simulink model "VCU_Final_Rev5"  (R2019b)
settings: Solver=FixedStepDiscrete  StartTime=0.0  StopTime=10.0  FixedStep=0.001  RelTol=1e-3  EnableMultiTasking=on
InitFcn:
  | EcoCoder_PreCheckLic();
libraries: CoderSF_BSW_Libs x68, SF_CanService_Libs x13
settings Model: Creator=andif  LastModifiedBy=andif
settings DataIOCC: SaveFormat=Structure  SignalLoggingSaveFormat=ModelDataLogs  SaveOutput=off  SignalLogging=off  DSMLogging=off  SaveTime=off  ReturnWorkspaceOutputs=off
settings OptimizationCC: DefaultParameterBehavior=Inlined  InlineInvariantSignals=on  EnhancedBackFolding=on  StrengthReduction=on  EnableMemcpy=off  PassReuseOutputArgsAs=Individual arguments  EfficientFloat2IntCast=on  LifeSpan=1  SimCompilerOptimization=on  OptimizeBlockOrder=speed  DifferentSizesBufferReuse=on  EfficientTunableParamExpr=on
settings DebuggingCC: AlgebraicLoopMsg=none  ArtificialAlgebraicLoopMsg=none  SaveWithDisabledLinksMsg=none  SaveWithParameterizedLinksMsg=none  CheckSSInitialOutputMsg=off  UnderspecifiedInitializationDetection=Classic  SignalResolutionControl=TryResolveAll  BlockPriorityViolationMsg=error  MinStepSizeMsg=none  InheritedTsInSrcMsg=none  MultiTaskDSMMsg=none  MultiTaskCondExecSysMsg=none  MultiTaskRateTransMsg=warning  TasksWithSamePriorityMsg=none  SigSpecEnsureSampleTimeMsg=none  IntegerOverflowMsg=error  Int32ToFloatConvMsg=none  ParameterPrecisionLossMsg=none  ParameterTunabilityLossMsg=none  FixptConstOverflowMsg=error  FcnCallInpInsideContextMsg=warning  UnconnectedInputMsg=error  UnconnectedOutputMsg=error  UnconnectedLineMsg=error  FrameProcessingCompatibilityMsg=none  BusObjectLabelMismatch=none  RootOutportRequireBusObject=none  UnknownTsInhSupMsg=none  ModelReferenceDataLoggingMessage=none  SFUnusedDataAndEventsDiag=none  SFUnexpectedBacktrackingDiag=none  SFInvalidInputDataAccessInChartInitDiag=none  SFNoUnconditionalDefaultTransitionDiag=none  SFTransitionOutsideNaturalParentDiag=none  SFUnreachableExecutionPathDiag=none
settings HardwareCC: ProdBitPerPointer=32  ProdBitPerSizeT=32  ProdBitPerPtrDiffT=32  ProdLargestAtomicInteger=Long  ProdLargestAtomicFloat=Double  ProdEndianess=BigEndian  ProdWordSize=32  ProdHWDeviceType=Freescale->MPC55xx
settings ModelReferenceCC: UpdateModelReferenceTargets=Force  ModelReferenceNumInstancesAllowed=Single  PropagateSignalLabelsOutOfModel=off
settings SFSimCC: SFSimEcho=off  SimBuildMode=sf_make_clean  MATLABDynamicMemAlloc=off
settings RTWCC: Description=Ecotrons MPC5xxx  SystemTargetFile=MPC5644A.tlc  GenerateMakefile=off  TemplateMakefile=ert_default_tmf  RTWVerbose=off  RetainRTWFile=on  RTWCompilerOptimization=on
settings CodeAppCC: IgnoreCustomStorageClasses=off  OperatorAnnotations=on  CustomSymbolStrGlobalVar=$N$M  CustomSymbolStrType=$N$M  CustomSymbolStrFcn=$N$M  CustomSymbolStrFcnArg=$N$M  CustomSymbolStrBlkIO=$N$M  CustomSymbolStrMacro=$N$M
settings STFCustomTargetCC: TargetLangStandard=C99 (ISO)  CodeReplacementLibrary=ANSI_C  UtilityFuncGeneration=Shared location  MultiwordLength=256  IncludeMdlTerminateFcn=off  CombineOutputUpdateFcns=on  SuppressErrorStatus=on  ERTCustomFileBanners=on  SupportNonFinite=off  SupportComplex=off  SupportContinuousTime=off  SupportNonInlinedSFcns=off  MATLABClassNameForMDSCustomization=Simulink.SoftwareTarget.ERTCustomization  SystemTargetFile=MPC5644A.tlc
settings ERTTargetCC: TargetLangStandard=C99 (ISO)  CodeReplacementLibrary=ANSI_C  UtilityFuncGeneration=Shared location  ParMdlRefBuildCompliant=off  CompOptLevelCompliant=off  ConcurrentExecutionCompliant=off  IncludeMdlTerminateFcn=off  SuppressErrorStatus=on  SupportNonFinite=off  SupportComplex=off  RemoveResetFunc=off  ModelStepFunctionPrototypeControlCompliant=off  CPPClassGenCompliant=off  UseToolchainInfoCompliant=off  GenerateASAP2=on  InlinedParameterPlacement=NonHierarchical  ERTCustomFileTemplate=MPC5644A_file_process.tlc  ERTFilePackagingFormat=Compact  PreserveIfCondition=on  ConvertIfToSwitch=off  PreserveExternInFcnDecls=off  SuppressUnreachableDefaultCases=off

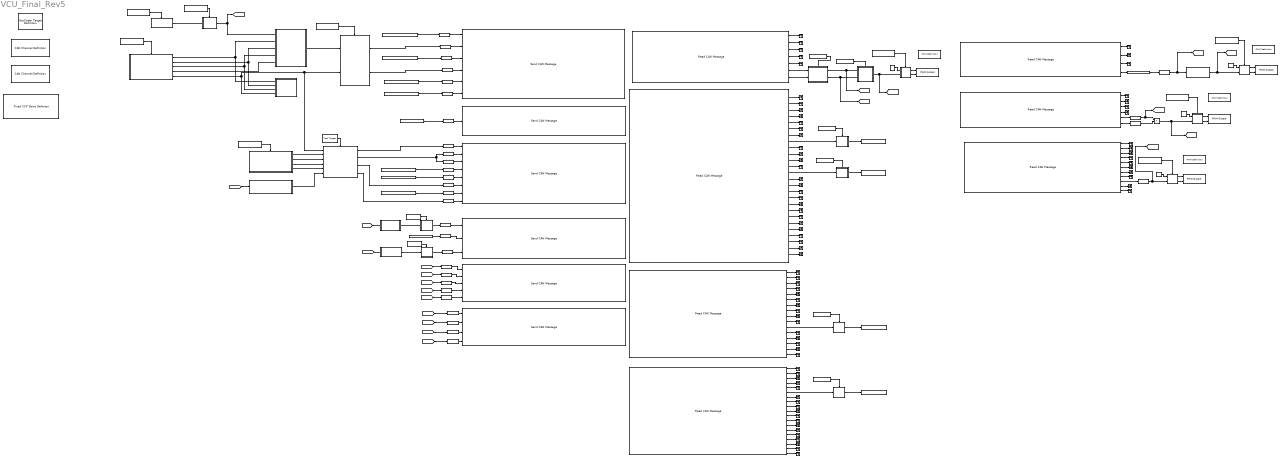
== system VCU_Final_Rev5 ==
  note: Get Power
  note: Speed2PWM. 0-10000RPM = 0-100% duty cycle, 488Hz
  note: SOC2PWM. 0-100% = 0-100% duty cycle, 488Hz
  note: CHGPOW2PWM. 0-10000W = 0-100% duty cycle, 488Hz
  note: MotPow2PWM. 0-100kW = 0-100% duty cycle, 488Hz
  CAN Channel Definition : CoderSF_BSW_Libs/CAN/CAN Channel Definition  channel=CAN_A  can_en=on  can_idfilter=off  can_rxextended=off  can_rxMask=hex2dec('7ff')  can_rxID=hex2dec('100')  can_baudrateIndex=500  can_txbuffer_size=30  can_rxbuffer_size=1  can_en_fd=off  nominalSamplePoint=7500  can_baudrateIndex_data=500  fastSamplePoint=7500  canfd_txbuffer_size=5  EcoCoderBlockID=C001_CANDef
  CAN Channel Definition1 : CoderSF_BSW_Libs/CAN/CAN Channel Definition  channel=CAN_C  can_en=on  can_idfilter=off  can_rxextended=off  can_rxMask=hex2dec('7ff')  can_rxID=hex2dec('100')  can_baudrateIndex=500  can_txbuffer_size=30  can_rxbuffer_size=1  can_en_fd=off  nominalSamplePoint=7500  can_baudrateIndex_data=500  fastSamplePoint=7500  canfd_txbuffer_size=5  EcoCoderBlockID=C001_CANDef
  ChgControl : Subsystem
  ChgCutOff : Subsystem
  Constant{,1..3} (4 alike) : Constant  Value=488
  Convert : Subsystem
  Data Type Conversion{,1..30} (31 alike) : DataTypeConversion
  Driver Input : Subsystem
  EcoCoder Target Definition : CoderSF_BSW_Libs/EcoCoder Target Definition  targetECU=EV2106B01  EcoCoderBlockID=T001_Target  enNoTriggerCall=on  flgBlockReduction=on  flgShowDebugDisp=off  flgDisTargetOutFIleCounter=off  flgClearAllOldFiles=on  tc275_cal_len=hex2dec('00008000')  internal_flash=[hex2dec('00020000'),hex2dec('000E0000')]  cal_rom_phy=[hex2dec('00010000'),hex2dec('00002000')]  cal_ram_wp=[hex2dec('4000F000'),hex2dec('00002000')]  cal_ram_msm=[hex2dec('40000000'),hex2dec('00002000')]  var_ram_wp=[hex2dec('40002000'),hex2dec('0000D000')]  write_back_fixed_ram=[hex2dec('40011000'),hex2dec('00001000')]  write_back_unfixed_ram=[hex2dec('40012000'),hex2dec('00001000')]  stack=[hex2dec('40013000'),hex2dec('00001000')]
      settings: AttributesFormatString=Target :%<targetECU>
  Fixed CCP Slave Definiton : CoderSF_BSW_Libs/CCP/Fixed CCP Slave Definiton  ccpType=Configurable  ccp_enSet=on  ccp_disASW=on  channel=CAN_C  stationaddressSet=hex2dec('0112')  croidSet=hex2dec('100')  dtoidSet=hex2dec('101')  daqidSet=[hex2dec('101') hex2dec('101') hex2dec('101') hex2dec('102')]  daqpidSet=[hex2dec('0') hex2dec('3C') hex2dec('78') hex2dec('0')]  daqlenSet=[hex2dec('0') hex2dec('20') hex2dec('30') hex2dec('30')]  daqperSet=[5 20 100 0]  EcoCoderBlockID=C002_CCPConf
  GetMotPower : Subsystem
  OBCInputCheck : Subsystem
  Output_Interface : Subsystem
  PWM Definition : CoderSF_BSW_Libs/Digital I//O/PWM Definition  EcoCoderBlockID=D001_OPWMDef  channel=LSO14  opwm_en=on  opwm_freq=488  opwm_duty=0
  PWM Definition1 : CoderSF_BSW_Libs/Digital I//O/PWM Definition  EcoCoderBlockID=D001_OPWMDef  channel=LSO16  opwm_en=on  opwm_freq=488  opwm_duty=0
  PWM Definition2 : CoderSF_BSW_Libs/Digital I//O/PWM Definition  EcoCoderBlockID=D001_OPWMDef  channel=HSO11  opwm_en=on  opwm_freq=488  opwm_duty=0
  PWM Definition3 : CoderSF_BSW_Libs/Digital I//O/PWM Definition  EcoCoderBlockID=D001_OPWMDef  channel=HSO12  opwm_en=on  opwm_freq=488  opwm_duty=0
  PWM Output : CoderSF_BSW_Libs/Digital I//O/PWM Output  channel=HSO11
  PWM Output1 : CoderSF_BSW_Libs/Digital I//O/PWM Output  channel=HSO12
  PWM Output2 : CoderSF_BSW_Libs/Digital I//O/PWM Output  channel=LSO16
  PWM Output3 : CoderSF_BSW_Libs/Digital I//O/PWM Output  channel=LSO14
  ParkMode : Subsystem
  PedalInput : Subsystem
  PowerTrain : Subsystem
  Product : Product
  Read CAN Message : SF_CanService_Libs/Read CAN Message  typeCAN=Connected  channel=CAN_A  mEn=off  msgInfo=MCU  msgIterm=MCU_State_1  msgItermStore=MCU_State_1  valid=on  stale=on  motoBit=off  setSignalName=off  flgCustomMonitorVariableRules=on  defineSignalName=off  prefixSignal='rxCANABMS'  flgValTest=off  flgNoFixed=on  tSample=Task_L10ms  modeCode=Parameterless
  Read CAN Message1 : SF_CanService_Libs/Read CAN Message  typeCAN=Connected  channel=CAN_A  mEn=off  msgInfo=OBCDCDC  msgIterm=DCDC_state_1  msgItermStore=DCDC_state_1  valid=on  stale=on  motoBit=off  setSignalName=off  flgCustomMonitorVariableRules=on  defineSignalName=off  prefixSignal='rxCANABMS'  flgValTest=off  flgNoFixed=on  tSample=Task_L100ms  modeCode=Parameterless
  Read CAN Message2 : SF_CanService_Libs/Read CAN Message  typeCAN=Connected  channel=CAN_A  mEn=off  msgInfo=MCU  msgIterm=MCU_Faliure_1  msgItermStore=MCU_Faliure_1  valid=on  stale=on  motoBit=off  setSignalName=off  flgCustomMonitorVariableRules=on  defineSignalName=off  prefixSignal='rxCANABMS'  flgValTest=off  flgNoFixed=on  tSample=Task_L100ms  modeCode=Parameterless
  Read CAN Message3 : SF_CanService_Libs/Read CAN Message  typeCAN=Connected  channel=CAN_A  mEn=off  msgInfo=OBCDCDC  msgIterm=OBC_state_1  msgItermStore=OBC_state_1  valid=on  stale=on  motoBit=off  setSignalName=off  flgCustomMonitorVariableRules=on  defineSignalName=off  prefixSignal='rxCANABMS'  flgValTest=off  flgNoFixed=on  tSample=Task_L100ms  modeCode=Parameterless
  Read CAN Message5 : SF_CanService_Libs/Read CAN Message  typeCAN=Connected  channel=CAN_A  mEn=off  msgInfo=OBCDCDC  msgIterm=HCM_state_4  msgItermStore=HCM_state_4  valid=on  stale=on  motoBit=off  setSignalName=off  flgCustomMonitorVariableRules=on  defineSignalName=off  prefixSignal='rxCANABMS'  flgValTest=off  flgNoFixed=on  tSample=Task_L20ms  modeCode=Parameterless
  Read CAN Message6 : SF_CanService_Libs/Read CAN Message  typeCAN=Connected  channel=CAN_A  mEn=off  msgInfo=OBCDCDC  msgIterm=OBC_state_2  msgItermStore=OBC_state_2  valid=on  stale=on  motoBit=off  setSignalName=off  flgCustomMonitorVariableRules=on  defineSignalName=off  prefixSignal='rxCANABMS'  flgValTest=off  flgNoFixed=on  tSample=Task_L20ms  modeCode=Parameterless
  Read CAN Message7 : SF_CanService_Libs/Read CAN Message  typeCAN=Connected  channel=CAN_A  mEn=off  msgInfo=MCU  msgIterm=MCU_State_2  msgItermStore=MCU_State_2  valid=on  stale=on  motoBit=off  setSignalName=off  flgCustomMonitorVariableRules=on  defineSignalName=off  prefixSignal='rxCANABMS'  flgValTest=off  flgNoFixed=on  tSample=Task_L10ms  modeCode=Parameterless
  Read Calibration1 : CoderSF_BSW_Libs/Calibration & Measurement/Read Calibration  variable_name=txCMD_HCM_shutsdown_hibernation_val  variable_value=0  variable_type=single  variable_min=[]  variable_max=[]  unitStr=""  descStr=""
      settings: AttributesFormatString=value:%<variable_value> type:%<variable_type> max:%<variable_max> Min:%<variable_min>
  Read Calibration2 : CoderSF_BSW_Libs/Calibration & Measurement/Read Calibration  variable_name=txCMD_HCM_shutsdown_hibernation_val  variable_value=0  variable_type=single  variable_min=[]  variable_max=[]  unitStr=""  descStr=""
      settings: AttributesFormatString=value:%<variable_value> type:%<variable_type> max:%<variable_max> Min:%<variable_min>
  Read Calibration3 : CoderSF_BSW_Libs/Calibration & Measurement/Read Calibration  variable_name=txCMD_Quick_Charge_Con_val  variable_value=1  variable_type=single  variable_min=[]  variable_max=[]  unitStr=""  descStr=""
      settings: AttributesFormatString=value:%<variable_value> type:%<variable_type> max:%<variable_max> Min:%<variable_min>
  Read Calibration6 : CoderSF_BSW_Libs/Calibration & Measurement/Read Calibration  variable_name=Running_mode  variable_value=0  variable_type=single  variable_min=[]  variable_max=[]  unitStr=""  descStr=""
      settings: AttributesFormatString=value:%<variable_value> type:%<variable_type> max:%<variable_max> Min:%<variable_min>
  Read Calibration7 : CoderSF_BSW_Libs/Calibration & Measurement/Read Calibration  variable_name=Motor_Direction  variable_value=0  variable_type=single  variable_min=[]  variable_max=[]  unitStr=""  descStr=""
      settings: AttributesFormatString=value:%<variable_value> type:%<variable_type> max:%<variable_max> Min:%<variable_min>
  Read Calibration8 : CoderSF_BSW_Libs/Calibration & Measurement/Read Calibration  variable_name=Motor_Speed  variable_value=0  variable_type=single  variable_min=[]  variable_max=[]  unitStr=""  descStr=""
      settings: AttributesFormatString=value:%<variable_value> type:%<variable_type> max:%<variable_max> Min:%<variable_min>
  Read Calibration9 : CoderSF_BSW_Libs/Calibration & Measurement/Read Calibration  variable_name=Motor_Control_Mode  variable_value=1  variable_type=boolean  variable_min=[]  variable_max=[]  unitStr=""  descStr=""
      settings: AttributesFormatString=value:%<variable_value> type:%<variable_type> max:%<variable_max> Min:%<variable_min>
  "Send CAN Message " : SF_CanService_Libs/Send CAN Message   typeCAN=Connected  channel=CAN_A  mEn=off  msgInfo=ALL  msgIterm=VCU_Transmit  msgItermStore=VCU_Transmit  motoBit=off  flgNoFixed=on  tSample=Task_L10ms  modeCode=Parameterless
  Send CAN Message 1 : SF_CanService_Libs/Send CAN Message   typeCAN=Connected  channel=CAN_A  mEn=off  msgInfo=OBCDCDC  msgIterm=CMD_2_VCU  msgItermStore=CMD_2_VCU  motoBit=off  flgNoFixed=on  tSample=Task_L50ms  modeCode=Parameterless
  Send CAN Message 2 : SF_CanService_Libs/Send CAN Message   typeCAN=Connected  channel=CAN_A  mEn=off  msgInfo=OBCDCDC  msgIterm=CMD_1_VCU  msgItermStore=CMD_1_VCU  motoBit=off  flgNoFixed=on  tSample=Task_L50ms  modeCode=Parameterless
  Send CAN Message 3 : SF_CanService_Libs/Send CAN Message   typeCAN=Connected  channel=CAN_A  mEn=off  msgInfo=OBCDCDC  msgIterm=CMD_4_BMS  msgItermStore=CMD_4_BMS  motoBit=off  flgNoFixed=on  tSample=Task_L50ms  modeCode=Parameterless
  Send CAN Message 4 : SF_CanService_Libs/Send CAN Message   typeCAN=Connected  channel=CAN_A  mEn=off  msgInfo=ALL  msgIterm=DATA_OUT2  msgItermStore=DATA_OUT2  motoBit=off  flgNoFixed=on  tSample=Task_L50ms  modeCode=Parameterless
  Send CAN Message 5 : SF_CanService_Libs/Send CAN Message   typeCAN=Connected  channel=CAN_A  mEn=off  msgInfo=ALL  msgIterm=DATA_OUT1  msgItermStore=DATA_OUT1  motoBit=off  flgNoFixed=on  tSample=Task_L50ms  modeCode=Parameterless
  Subsystem : Subsystem
  Subsystem1 : Subsystem
  Subsystem10 : Subsystem
  Subsystem11 : Subsystem
  Subsystem12 : Subsystem
  Subsystem13 : Subsystem
  Subsystem2 : Subsystem
  Subsystem3 : Subsystem
  Subsystem4 : Subsystem
  Subsystem7 : Subsystem
  Switch Output : CoderSF_BSW_Libs/Digital I//O/Switch Output  channel=LSO01
  Switch Output1 : CoderSF_BSW_Libs/Digital I//O/Switch Output  channel=LSO02
  Switch Output2 : CoderSF_BSW_Libs/Digital I//O/Switch Output  channel=LSO03
  Switch Output3 : CoderSF_BSW_Libs/Digital I//O/Switch Output  channel=LSO04
  Switching : Subsystem
  System Input : Subsystem
  Task_Call : CoderSF_BSW_Libs/Task Scheduler/Task Trigger  tasktimeIndex=Task_H10ms
  Task_Call{1..3,9,20..22} (7 alike) : CoderSF_BSW_Libs/Task Scheduler/Task Trigger  tasktimeIndex=Task_L10ms
  Task_Call{7..8,10..11} (4 alike) : CoderSF_BSW_Libs/Task Scheduler/Task Trigger  tasktimeIndex=Task_L100ms
  Task_Call13 : CoderSF_BSW_Libs/Task Scheduler/Task Trigger  tasktimeIndex=Task_L20ms
  Task_Call17 : CoderSF_BSW_Libs/Task Scheduler/Task Trigger  tasktimeIndex=Task_L20ms
  Task_Call{4..6,18} (4 alike) : CoderSF_BSW_Libs/Task Scheduler/Task Trigger  tasktimeIndex=Task_L50ms
  Terminator{,1..41,43..67,94..105} (79 alike) : Terminator
  Volt2SOC : Subsystem
  Write and Read Measurement2 : CoderSF_BSW_Libs/Calibration & Measurement/Write and Read Measurement  variable_name=Batt  variable_value=0  variable_type=uint16  numD=1  unitStr=""  descStr=""
      settings: AttributesFormatString=type:%<variable_type> Dimensions:%<numD>
  ecocoder_calibration1 : CoderSF_BSW_Libs/Calibration & Measurement/Read Calibration  variable_name=Chg_Cv  variable_value=400  variable_type=single  variable_min=[]  variable_max=[]  unitStr=""  descStr=""
      settings: AttributesFormatString=value:%<variable_value> type:%<variable_type> max:%<variable_max> Min:%<variable_min>
  ecocoder_calibration10 : CoderSF_BSW_Libs/Calibration & Measurement/Read Calibration  variable_name=Heartbeat  variable_value=1  variable_type=uint8  variable_min=[]  variable_max=[]  unitStr=""  descStr=""
      settings: AttributesFormatString=value:%<variable_value> type:%<variable_type> max:%<variable_max> Min:%<variable_min>
  volt2percent : Subsystem
  wires:
  Task_Call/1 -> PedalInput/Trigger
  ParkMode/2(Motor_en) -> Data Type Conversion3/1
  Driver Input/3(SportOut) -> PowerTrain/4(Sport), Output_Interface/3(SportLED)
  Driver Input/1(SwitchDOut) -> PowerTrain/2(Drive), Output_Interface/1(DriveLED)
  Data Type Conversion/1 -> "Send CAN Message "/2
  Data Type Conversion1/1 -> "Send CAN Message "/1
  Data Type Conversion5/1 -> "Send CAN Message "/6
  Data Type Conversion4/1 -> "Send CAN Message "/5
  Data Type Conversion3/1 -> "Send CAN Message "/4
  Data Type Conversion2/1 -> "Send CAN Message "/3
  PedalInput/1(sigInLinkDrvPedacc_volt1) -> volt2percent/1(In1)
  Task_Call1/1 -> volt2percent/Trigger
  Task_Call2/1 -> Driver Input/Trigger
  volt2percent/1(Out1) -> [ThrottlePCT], PowerTrain/1(Throttle)
  Driver Input/2(SwitchROut) -> PowerTrain/3(Reverse), Output_Interface/2(ReverseLED)
  Task_Call3/1 -> ParkMode/Trigger
  ParkMode/1(torque_Req) -> Data Type Conversion/1
  Task_Call4/1 -> System Input/Trigger
  Data Type Conversion8/1 -> Send CAN Message 1/3
  Data Type Conversion10/1 -> Send CAN Message 1/5
  Data Type Conversion9/1 -> Send CAN Message 1/4
  Data Type Conversion11/1 -> Send CAN Message 1/6
  Data Type Conversion13/1 -> Send CAN Message 1/8
  Data Type Conversion6/1 -> Send CAN Message 1/1
  Data Type Conversion12/1 -> Send CAN Message 1/7
  Data Type Conversion7/1 -> Send CAN Message 1/2
  Read Calibration2/1 -> Data Type Conversion9/1
  Read Calibration1/1 -> Data Type Conversion10/1
  Switching/3(OBC_out) -> Data Type Conversion11/1
  Read Calibration3/1 -> Data Type Conversion12/1
  Data Type Conversion14/1 -> Send CAN Message 2/1
  ecocoder_calibration10/1 -> Data Type Conversion14/1
  Task_Call5/1 -> Switching/Trigger
  Switching/1(Main_out) -> Data Type Conversion6/1
  Switching/2(AC_out) -> Data Type Conversion7/1, Data Type Conversion8/1
  Switching/4(DCDC_out) -> Data Type Conversion13/1
  Read Calibration6/1 -> Data Type Conversion5/1
  Read Calibration7/1 -> Data Type Conversion2/1
  Read Calibration8/1 -> Data Type Conversion1/1
  Read Calibration9/1 -> Data Type Conversion4/1
  Constant/1 -> Subsystem1/1(In1)
  Data Type Conversion21/1 -> [motSpeed], Subsystem1/2(In2)
  Subsystem1/1(Out1) -> PWM Output/1
  Subsystem1/2(Out2) -> PWM Output/2
  Task_Call9/1 -> Subsystem1/Trigger
  Read CAN Message2/5 -> Terminator41/1
  Read CAN Message2/4 -> Terminator40/1
  Read CAN Message2/3 -> Terminator39/1
  Read CAN Message2/2 -> Terminator38/1
  Read CAN Message2/1 -> Terminator37/1
  Read CAN Message2/10 -> Terminator47/1
  Read CAN Message/1 -> Terminator/1
  Read CAN Message/2 -> Terminator17/1
  Read CAN Message/3 -> Terminator49/1
  Read CAN Message/4 -> Terminator51/1
  Read CAN Message/5 -> Terminator50/1
  Read CAN Message/6 -> Terminator52/1
  Read CAN Message/7 -> Terminator53/1
  Read CAN Message/8 -> Terminator54/1
  Read CAN Message/10 -> Terminator55/1
  Read CAN Message/11 -> Terminator56/1
  Read CAN Message2/6 -> Terminator44/1
  Read CAN Message2/7 -> Terminator45/1
  Read CAN Message2/9 -> Terminator46/1
  Read CAN Message2/11 -> Terminator16/1
  Read CAN Message2/12 -> Terminator18/1
  Read CAN Message2/14 -> Terminator1/1
  Read CAN Message2/15 -> Terminator2/1
  Read CAN Message2/26 -> Terminator13/1
  Read CAN Message2/25 -> Terminator12/1
  Read CAN Message2/24 -> Terminator11/1
  Read CAN Message2/16 -> Terminator3/1
  Read CAN Message2/17 -> Terminator4/1
  Read CAN Message2/18 -> Terminator5/1
  Read CAN Message2/19 -> Terminator6/1
  Read CAN Message2/20 -> Terminator7/1
  Read CAN Message2/21 -> Terminator8/1
  Read CAN Message2/22 -> Terminator9/1
  Read CAN Message2/23 -> Terminator10/1
  ecocoder_calibration1/1 -> Data Type Conversion19/1
  Data Type Conversion19/1 -> Send CAN Message 3/2
  Driver Input/5(ParkOut) -> Switching/1(Park_in), ParkMode/2(park_in), Output_Interface/4(ParkLED)
  Read CAN Message1/1 -> Terminator14/1
  Read CAN Message1/2 -> Terminator15/1
  Read CAN Message1/3 -> Terminator19/1
  Read CAN Message1/4 -> Terminator20/1
  Read CAN Message1/16 -> Terminator32/1
  Read CAN Message1/15 -> Terminator31/1
  Read CAN Message1/14 -> Terminator30/1
  Read CAN Message1/13 -> Terminator29/1
  Read CAN Message1/12 -> Terminator28/1
  Read CAN Message1/10 -> Terminator26/1
  Read CAN Message1/9 -> Terminator25/1
  Read CAN Message1/8 -> Terminator24/1
  Read CAN Message1/7 -> Terminator23/1
  Read CAN Message1/6 -> Terminator22/1
  Read CAN Message1/5 -> Terminator21/1
  Read CAN Message2/8 -> Subsystem/1(In1)
  Subsystem/1(Out1) -> Switch Output/1
  Read CAN Message2/13 -> Subsystem2/1(In1)
  Subsystem2/1(Out1) -> Switch Output1/1
  Task_Call7/1 -> Subsystem/Trigger
  Task_Call8/1 -> Subsystem2/Trigger
  Subsystem3/1(Out1) -> Switch Output2/1
  Read CAN Message1/11 -> Subsystem3/1(In1)
  Task_Call10/1 -> Subsystem3/Trigger
  Read CAN Message3/1 -> Terminator27/1
  Read CAN Message3/2 -> Terminator33/1
  Read CAN Message3/3 -> Terminator34/1
  Read CAN Message3/4 -> Terminator35/1
  Read CAN Message3/5 -> Terminator36/1
  Read CAN Message3/7 -> Terminator43/1
  Read CAN Message3/8 -> Terminator48/1
  Read CAN Message3/9 -> Terminator57/1
  Read CAN Message3/10 -> Terminator58/1
  Read CAN Message3/11 -> Terminator59/1
  Read CAN Message3/12 -> Terminator60/1
  Read CAN Message3/13 -> Terminator61/1
  Read CAN Message3/14 -> Terminator62/1
  Read CAN Message3/15 -> Terminator63/1
  Read CAN Message3/16 -> Terminator64/1
  Read CAN Message3/17 -> Terminator65/1
  Read CAN Message3/18 -> Terminator66/1
  Read CAN Message3/19 -> Terminator67/1
  Task_Call11/1 -> Subsystem4/Trigger
  Subsystem4/1(Out1) -> Switch Output3/1
  Read CAN Message3/6 -> Subsystem4/1(In1)
  Read CAN Message5/2 -> Terminator96/1
  Read CAN Message5/1 -> Terminator94/1
  Read CAN Message5/3 -> Terminator95/1
  Read CAN Message5/4 -> Write and Read Measurement2/1
  Task_Call13/1 -> Subsystem7/Trigger
  Constant1/1 -> Subsystem7/1(In1)
  Subsystem7/2(Out2) -> PWM Output1/2
  Subsystem7/1(Out1) -> PWM Output1/1
  Volt2SOC/1(SOC) -> [SOC], Subsystem7/2(In2)
  Read CAN Message6/1 -> Terminator97/1
  Read CAN Message6/2 -> Terminator99/1
  Read CAN Message6/6 -> Data Type Conversion20/1
  Product/1 -> [OBCInPow], Subsystem10/2(In2)
  Subsystem10/2(Out2) -> PWM Output2/2
  Subsystem10/1(Out1) -> PWM Output2/1
  Constant2/1 -> Subsystem10/1(In1)
  Read CAN Message6/3 -> Terminator98/1
  Read CAN Message6/4 -> Terminator100/1
  Read CAN Message6/5 -> Data Type Conversion18/1
  Task_Call17/1 -> Subsystem10/Trigger
  Convert/1(Out1) -> Data Type Conversion15/1
  Task_Call18/1 -> Convert/Trigger
  Read CAN Message7/6 -> Subsystem11/1(MotACVoltRaw)
  Read CAN Message7/7 -> Subsystem11/2(MotACCurRaw)
  Read CAN Message/9 -> Data Type Conversion21/1
  Read CAN Message7/1 -> Terminator101/1
  Read CAN Message7/2 -> Terminator102/1
  Read CAN Message7/3 -> Terminator103/1
  Read CAN Message7/4 -> Terminator104/1
  Read CAN Message7/5 -> Terminator105/1
  Task_Call20/1 -> Subsystem11/Trigger
  Task_Call21/1 -> Subsystem12/Trigger
  Constant3/1 -> Subsystem12/1(In1)
  Subsystem12/2(Out2) -> PWM Output3/2
  Subsystem12/1(Out1) -> PWM Output3/1
  Subsystem11/1(MotACVolt) -> [motACVolt], GetMotPower/1(MotVolt)
  Subsystem11/2(MotACCur) -> [motACCur], GetMotPower/2(MotCur)
  GetMotPower/1(MotPow) -> [motPow], Subsystem12/2(In2)
  Task_Call22/1 -> GetMotPower/Trigger
  Subsystem13/1(Out1) -> Data Type Conversion17/1
  Task_Call6/1 -> Subsystem13/Trigger
  Data Type Conversion15/1 -> Send CAN Message 3/1
  Data Type Conversion17/1 -> Send CAN Message 3/3
  Write and Read Measurement2/1 -> Data Type Conversion16/1  "Batt"
  ChgCutOff/1(Out1) -> Subsystem13/1(In1)
  System Input/1(OBC_Sw) -> Switching/2(OBC_in1)
  System Input/2(DCDC_Sw) -> Switching/3(DCDC_in2)  "DCDC_en"
  System Input/3(MAIN_Sw) -> Switching/4(Main_in)
  System Input/4(AC_Sw) -> Switching/5(AC_in)
  OBCInputCheck/1(Out1) -> Switching/6(ChgIn)
  Driver Input/4(BrakeOut) -> PowerTrain/5(brake_in)
  PowerTrain/1(TorqueRequest) -> ParkMode/1(Torque)
  Data Type Conversion16/1 -> [BattVolt], Volt2SOC/1(BattPackVoltage)
  Data Type Conversion20/1 -> Product/2
  ChgControl/1(Out1) -> Convert/1(In1)
  Data Type Conversion18/1 -> [OBCInVolt], Product/1
  Data Type Conversion23/1 -> Send CAN Message 4/3
  Data Type Conversion22/1 -> Send CAN Message 4/4
  Data Type Conversion24/1 -> Send CAN Message 4/2
  Data Type Conversion25/1 -> Send CAN Message 4/1
  [BattVolt] -> ChgControl/1(In1)
  [BattVolt] -> ChgCutOff/1(In1)
  [OBCInVolt] -> OBCInputCheck/1(In1)
  Data Type Conversion29/1 -> Send CAN Message 5/1
  Data Type Conversion28/1 -> Send CAN Message 5/2
  Data Type Conversion27/1 -> Send CAN Message 5/3
  Data Type Conversion26/1 -> Send CAN Message 5/4
  [motPow] -> Data Type Conversion29/1
  [motACVolt] -> Data Type Conversion28/1
  [motACCur] -> Data Type Conversion27/1
  [motSpeed] -> Data Type Conversion26/1
  [BattVolt] -> Data Type Conversion30/1
  Data Type Conversion30/1 -> Send CAN Message 4/5
  [OBCInVolt] -> Data Type Conversion22/1
  [SOC] -> Data Type Conversion23/1
  [ThrottlePCT] -> Data Type Conversion25/1
  [OBCInPow] -> Data Type Conversion24/1

== system VCU_Final_Rev5/ChgControl ==
  note: Batt Voltage & Current Plot for OBC
  In1 : Inport
  VoltageVSCurrent : CoderSF_BSW_Libs/Calibration & Measurement/1-D Lookup Table  nam=ChgControl  breakpoint_type=single  breakpoint_data=[0 200 220 250 260 280 300 320 330 400]  table_type=single  table_data=[18 18 18 18 20 20 20 20 20 0]
  Out1 : Outport
  wires:
  In1/1 -> VoltageVSCurrent/1
  VoltageVSCurrent/1 -> Out1/1

== system VCU_Final_Rev5/ChgCutOff ==
  note: If Batt >401VDC. send 1 to cut.
  In1 : Inport
  Constant4 : Constant
  Constant5 : Constant  Value=2
  Switch : Switch  Threshold=401
  Out1 : Outport
  wires:
  Constant4/1 -> Switch/1
  Switch/1 -> Out1/1
  In1/1 -> Switch/2
  Constant5/1 -> Switch/3

== system VCU_Final_Rev5/Convert ==
  In1 : Inport
  f : TriggerPort  TriggerType=function-call  VariantControl=(inherit)
  Data Type Conversion15 : DataTypeConversion
  Out1 : Outport
  wires:
  Data Type Conversion15/1 -> Out1/1
  In1/1 -> Data Type Conversion15/1

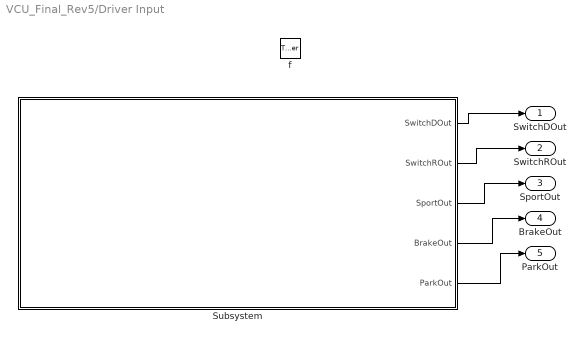
== system VCU_Final_Rev5/Driver Input ==
  f : TriggerPort  TriggerType=function-call  VariantControl=(inherit)
  Subsystem : Subsystem
  SwitchDOut : Outport
  SwitchROut : Outport  Port=2
  SportOut : Outport  Port=3
  BrakeOut : Outport  Port=4
  ParkOut : Outport  Port=5
  wires:
  Subsystem/1(SwitchDOut) -> SwitchDOut/1
  Subsystem/2(SwitchROut) -> SwitchROut/1
  Subsystem/3(SportOut) -> SportOut/1
  Subsystem/4(BrakeOut) -> BrakeOut/1
  Subsystem/5(ParkOut) -> ParkOut/1

== system VCU_Final_Rev5/GetMotPower ==
  note: Power = V*I. Convert Watt to kW
  MotVolt : Inport
  MotCur : Inport  Port=2
  f : TriggerPort  TriggerType=function-call  VariantControl=(inherit)
  Product1 : Product
  W2kW : Gain  Gain=1/1000
  MotPow : Outport
  wires:
  Product1/1 -> W2kW/1
  W2kW/1 -> MotPow/1
  MotVolt/1 -> Product1/1
  MotCur/1 -> Product1/2

== system VCU_Final_Rev5/OBCInputCheck ==
  note: If input voltage > 100VAC, send high
  In1 : Inport
  Constant4 : Constant
  Constant5 : Constant  Value=0
  Switch : Switch  Criteria=u2 > Threshold  Threshold=100
  Out1 : Outport
  wires:
  Constant4/1 -> Switch/1
  Switch/1 -> Out1/1
  In1/1 -> Switch/2
  Constant5/1 -> Switch/3

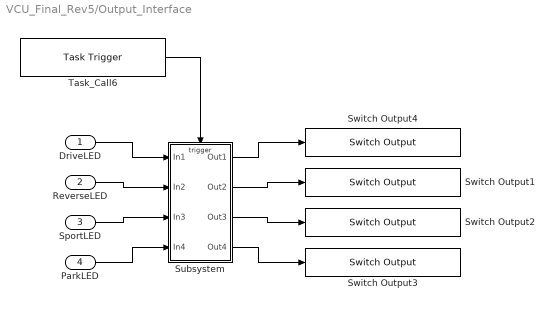
== system VCU_Final_Rev5/Output_Interface ==
  DriveLED : Inport
  ReverseLED : Inport  Port=2
  SportLED : Inport  Port=3
  ParkLED : Inport  Port=4
  Subsystem : Subsystem
  Switch Output1 : CoderSF_BSW_Libs/Digital I//O/Switch Output  channel=HSO14
  Switch Output2 : CoderSF_BSW_Libs/Digital I//O/Switch Output  channel=HSO15
  Switch Output3 : CoderSF_BSW_Libs/Digital I//O/Switch Output  channel=HSO16
  Switch Output4 : CoderSF_BSW_Libs/Digital I//O/Switch Output  channel=HSO13
  Task_Call6 : CoderSF_BSW_Libs/Task Scheduler/Task Trigger  tasktimeIndex=Task_L10ms
  wires:
  DriveLED/1 -> Subsystem/1(In1)
  ReverseLED/1 -> Subsystem/2(In2)
  SportLED/1 -> Subsystem/3(In3)
  ParkLED/1 -> Subsystem/4(In4)
  Subsystem/1(Out1) -> Switch Output4/1
  Subsystem/2(Out2) -> Switch Output1/1
  Subsystem/3(Out3) -> Switch Output2/1
  Subsystem/4(Out4) -> Switch Output3/1
  Task_Call6/1 -> Subsystem/Trigger

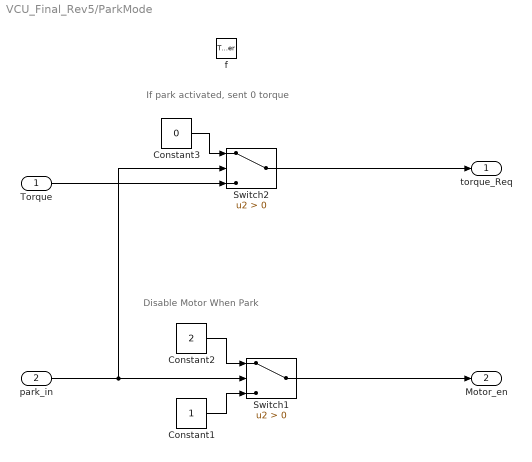
== system VCU_Final_Rev5/ParkMode ==
  note: If park activated, sent 0 torque
  note: Disable Motor When Park
  Torque : Inport
  park_in : Inport  Port=2
  f : TriggerPort  TriggerType=function-call  VariantControl=(inherit)
  Constant1 : Constant
  Constant2 : Constant  Value=2
  Constant3 : Constant  Value=0
  Switch1 : Switch  Criteria=u2 > Threshold
  Switch2 : Switch  Criteria=u2 > Threshold
  torque_Req : Outport
  Motor_en : Outport  Port=2
  wires:
  park_in/1 -> Switch2/2, Switch1/2
  Constant1/1 -> Switch1/3
  Constant2/1 -> Switch1/1
  Constant3/1 -> Switch2/1
  Switch2/1 -> torque_Req/1
  Switch1/1 -> Motor_en/1
  Torque/1 -> Switch2/3

== system VCU_Final_Rev5/PedalInput ==
  f : TriggerPort  TriggerType=function-call  VariantControl=(inherit)
  Subsystem : Subsystem
  sigInLinkDrvPedacc_volt1 : Outport
  wires:
  Subsystem/1(sigInLinkDrvPedacc_volt1) -> sigInLinkDrvPedacc_volt1/1

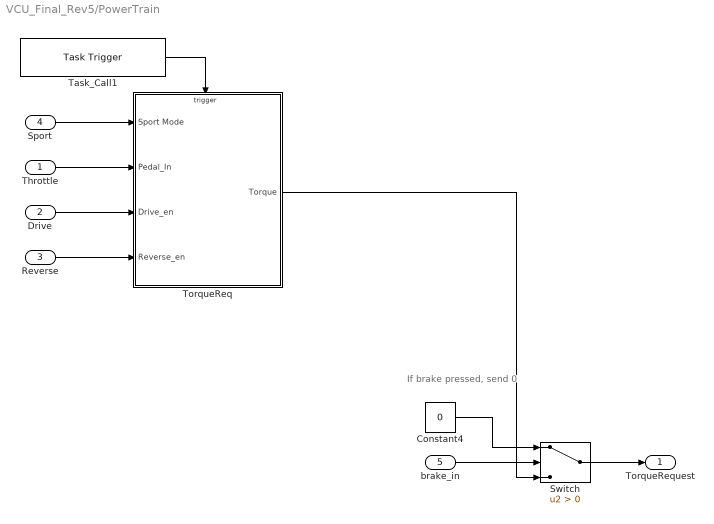
== system VCU_Final_Rev5/PowerTrain ==
  note: If brake pressed, send 0
  Throttle : Inport
  Drive : Inport  Port=2
  Reverse : Inport  Port=3
  Sport : Inport  Port=4
  brake_in : Inport  Port=5
  Constant4 : Constant  Value=0
  Switch : Switch  Criteria=u2 > Threshold
  Task_Call1 : CoderSF_BSW_Libs/Task Scheduler/Task Trigger  tasktimeIndex=Task_L10ms
  TorqueReq : Subsystem
  TorqueRequest : Outport
  wires:
  Sport/1 -> TorqueReq/1(Sport Mode)
  Throttle/1 -> TorqueReq/2(Pedal_In)
  Drive/1 -> TorqueReq/3(Drive_en)
  Reverse/1 -> TorqueReq/4(Reverse_en)
  Task_Call1/1 -> TorqueReq/Trigger
  Switch/1 -> TorqueRequest/1
  brake_in/1 -> Switch/2
  Constant4/1 -> Switch/1
  TorqueReq/1(Torque) -> Switch/3

== system VCU_Final_Rev5/Subsystem ==
  In1 : Inport
  f : TriggerPort  TriggerType=function-call  VariantControl=(inherit)
  Data Type Conversion16 : DataTypeConversion
  Out1 : Outport
  wires:
  In1/1 -> Data Type Conversion16/1
  Data Type Conversion16/1 -> Out1/1

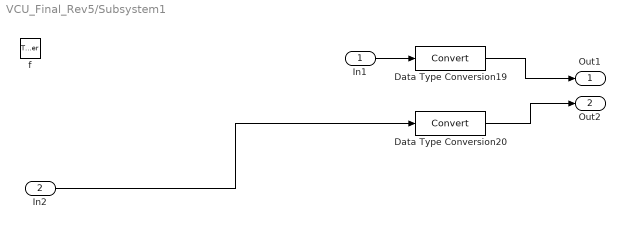
== system VCU_Final_Rev5/Subsystem1 ==
  In1 : Inport
  In2 : Inport  Port=2
  f : TriggerPort  TriggerType=function-call  VariantControl=(inherit)
  Data Type Conversion19 : DataTypeConversion
  Data Type Conversion20 : DataTypeConversion
  Out1 : Outport
  Out2 : Outport  Port=2
  wires:
  Data Type Conversion20/1 -> Out2/1
  In2/1 -> Data Type Conversion20/1
  Data Type Conversion19/1 -> Out1/1
  In1/1 -> Data Type Conversion19/1

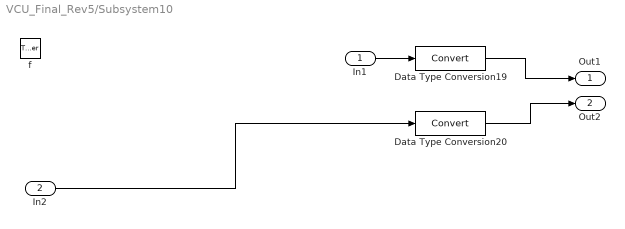
== system VCU_Final_Rev5/Subsystem10 ==
  In1 : Inport
  In2 : Inport  Port=2
  f : TriggerPort  TriggerType=function-call  VariantControl=(inherit)
  Data Type Conversion19 : DataTypeConversion
  Data Type Conversion20 : DataTypeConversion
  Out1 : Outport
  Out2 : Outport  Port=2
  wires:
  Data Type Conversion20/1 -> Out2/1
  In2/1 -> Data Type Conversion20/1
  Data Type Conversion19/1 -> Out1/1
  In1/1 -> Data Type Conversion19/1

== system VCU_Final_Rev5/Subsystem11 ==
  MotACVoltRaw : Inport
  MotACCurRaw : Inport  Port=2
  f : TriggerPort  TriggerType=function-call  VariantControl=(inherit)
  Data Type Conversion : DataTypeConversion
  Data Type Conversion1 : DataTypeConversion
  MotACVolt : Outport
  MotACCur : Outport  Port=2
  wires:
  Data Type Conversion/1 -> MotACVolt/1
  MotACVoltRaw/1 -> Data Type Conversion/1
  Data Type Conversion1/1 -> MotACCur/1
  MotACCurRaw/1 -> Data Type Conversion1/1

== system VCU_Final_Rev5/Subsystem12 ==
  In1 : Inport
  In2 : Inport  Port=2
  f : TriggerPort  TriggerType=function-call  VariantControl=(inherit)
  Data Type Conversion19 : DataTypeConversion
  Data Type Conversion20 : DataTypeConversion
  Out1 : Outport
  Out2 : Outport  Port=2
  wires:
  Data Type Conversion20/1 -> Out2/1
  In2/1 -> Data Type Conversion20/1
  Data Type Conversion19/1 -> Out1/1
  In1/1 -> Data Type Conversion19/1

== system VCU_Final_Rev5/Subsystem13 ==
  In1 : Inport
  f : TriggerPort  TriggerType=function-call  VariantControl=(inherit)
  Data Type Conversion17 : DataTypeConversion
  Out1 : Outport
  wires:
  In1/1 -> Data Type Conversion17/1
  Data Type Conversion17/1 -> Out1/1

== system VCU_Final_Rev5/Subsystem2 ==
  In1 : Inport
  f : TriggerPort  TriggerType=function-call  VariantControl=(inherit)
  Data Type Conversion15 : DataTypeConversion
  Out1 : Outport
  wires:
  In1/1 -> Data Type Conversion15/1
  Data Type Conversion15/1 -> Out1/1

== system VCU_Final_Rev5/Subsystem3 ==
  In1 : Inport
  f : TriggerPort  TriggerType=function-call  VariantControl=(inherit)
  Data Type Conversion15 : DataTypeConversion
  Out1 : Outport
  wires:
  In1/1 -> Data Type Conversion15/1
  Data Type Conversion15/1 -> Out1/1

== system VCU_Final_Rev5/Subsystem4 ==
  In1 : Inport
  f : TriggerPort  TriggerType=function-call  VariantControl=(inherit)
  Data Type Conversion15 : DataTypeConversion
  Out1 : Outport
  wires:
  In1/1 -> Data Type Conversion15/1
  Data Type Conversion15/1 -> Out1/1

== system VCU_Final_Rev5/Subsystem7 ==
  In1 : Inport
  In2 : Inport  Port=2
  f : TriggerPort  TriggerType=function-call  VariantControl=(inherit)
  Data Type Conversion19 : DataTypeConversion
  Data Type Conversion20 : DataTypeConversion
  Out1 : Outport
  Out2 : Outport  Port=2
  wires:
  Data Type Conversion20/1 -> Out2/1
  In2/1 -> Data Type Conversion20/1
  Data Type Conversion19/1 -> Out1/1
  In1/1 -> Data Type Conversion19/1

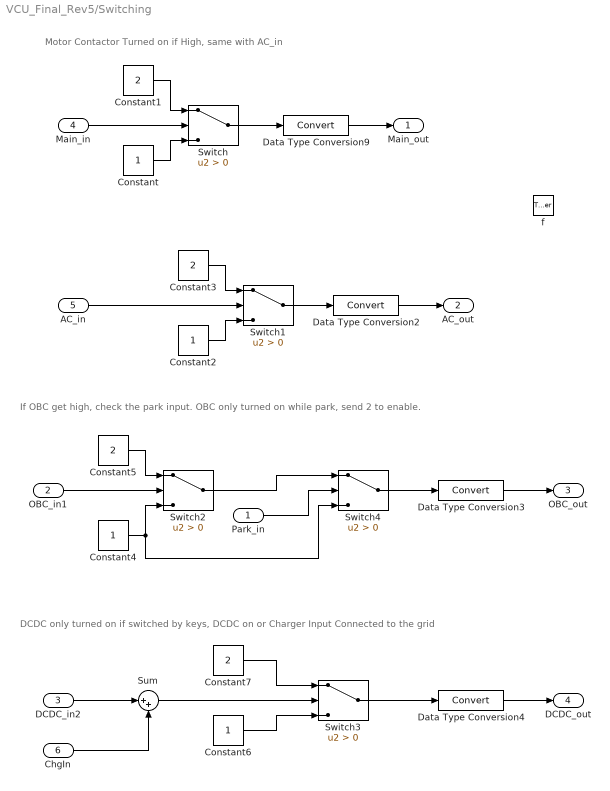
== system VCU_Final_Rev5/Switching ==
  note: If OBC get high, check the park input. OBC only turned on while park, send 2 to enable.
  note: Motor Contactor Turned on if High, same with AC_in
  note: DCDC only turned on if switched by keys, DCDC on or Charger Input Connected to the grid
  Park_in : Inport
  OBC_in1 : Inport  Port=2
  DCDC_in2 : Inport  Port=3
  Main_in : Inport  Port=4
  AC_in : Inport  Port=5
  ChgIn : Inport  Port=6
  f : TriggerPort  TriggerType=function-call  VariantControl=(inherit)
  Constant{,2,4,6} (4 alike) : Constant
  Constant{1,3,5,7} (4 alike) : Constant  Value=2
  Data Type Conversion{2..4,9} (4 alike) : DataTypeConversion
  Sum : Sum  Inputs=|++
  Switch{,1..4} (5 alike) : Switch  Criteria=u2 > Threshold
  Main_out : Outport
  AC_out : Outport  Port=2
  OBC_out : Outport  Port=3
  DCDC_out : Outport  Port=4
  wires:
  Data Type Conversion9/1 -> Main_out/1
  Data Type Conversion2/1 -> AC_out/1
  Data Type Conversion3/1 -> OBC_out/1
  Data Type Conversion4/1 -> DCDC_out/1
  Main_in/1 -> Switch/2
  Switch/1 -> Data Type Conversion9/1
  Constant1/1 -> Switch/1
  Constant/1 -> Switch/3
  AC_in/1 -> Switch1/2
  Switch1/1 -> Data Type Conversion2/1
  Constant2/1 -> Switch1/3
  Constant3/1 -> Switch1/1
  OBC_in1/1 -> Switch2/2
  Switch2/1 -> Switch4/1
  Constant4/1 -> Switch2/3, Switch4/3
  Constant5/1 -> Switch2/1
  Constant6/1 -> Switch3/3
  Constant7/1 -> Switch3/1
  Switch4/1 -> Data Type Conversion3/1
  Park_in/1 -> Switch4/2
  ChgIn/1 -> Sum/2
  Switch3/1 -> Data Type Conversion4/1
  DCDC_in2/1 -> Sum/1
  Sum/1 -> Switch3/2

== system VCU_Final_Rev5/System Input ==
  f : TriggerPort  TriggerType=function-call  VariantControl=(inherit)
  Subsystem : Subsystem
  OBC_Sw : Outport
  DCDC_Sw : Outport  Port=2
  MAIN_Sw : Outport  Port=3
  AC_Sw : Outport  Port=4
  wires:
  Subsystem/1(OBC_Sw) -> OBC_Sw/1
  Subsystem/2(DCDC_Sw) -> DCDC_Sw/1
  Subsystem/3(MAIN_Sw) -> MAIN_Sw/1
  Subsystem/4(AC_Sw) -> AC_Sw/1

== system VCU_Final_Rev5/Volt2SOC ==
  note: Limiter
  note: Voltage & SOC of the battery
  note: Divided to 96
      | to get cell voltage
  BattPackVoltage : Inport
  Bp2C : Gain  Gain=1/96
  CellVoltage2SOC : CoderSF_BSW_Libs/Calibration & Measurement/1-D Lookup Table  nam=SOC  breakpoint_type=single  breakpoint_data=|  table_type=single  table_data=|
      breakpoint_data=|
      | [3.036
      | 3.339
      | 3.477
      | 3.574
      | 3.638
      | 3.705
      | 3.823
      | 3.917
      | 4.014
      | 4.088
      | 4.164]
      table_data=|
      | [0
      | 10
      | 20
      | 30
      | 40
      | 50
      | 60
      | 70
      | 80
      | 90
      | 100]
  Saturation : Saturate  UpperLimit=100  LowerLimit=0
  SOC : Outport
  wires:
  CellVoltage2SOC/1 -> Saturation/1  "SOC"
  BattPackVoltage/1 -> Bp2C/1
  Bp2C/1 -> CellVoltage2SOC/1
  Saturation/1 -> SOC/1

== system VCU_Final_Rev5/volt2percent ==
  In1 : Inport
  f : TriggerPort  TriggerType=function-call  VariantControl=(inherit)
  Subsystem : Subsystem
  Out1 : Outport
  wires:
  In1/1 -> Subsystem/1(In1)
  Subsystem/1(Out1) -> Out1/1

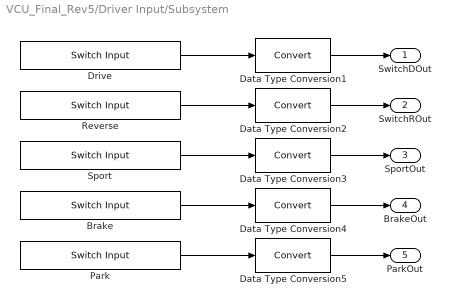
== system VCU_Final_Rev5/Driver Input/Subsystem ==
  Brake : CoderSF_BSW_Libs/Digital I//O/Switch Input  portNum=DI09
  Data Type Conversion{1..5} (5 alike) : DataTypeConversion
  Drive : CoderSF_BSW_Libs/Digital I//O/Switch Input  portNum=DI05
  Park : CoderSF_BSW_Libs/Digital I//O/Switch Input  portNum=DI08
  Reverse : CoderSF_BSW_Libs/Digital I//O/Switch Input  portNum=DI06
  Sport : CoderSF_BSW_Libs/Digital I//O/Switch Input  portNum=DI07
  SwitchDOut : Outport
  SwitchROut : Outport  Port=2
  SportOut : Outport  Port=3
  BrakeOut : Outport  Port=4
  ParkOut : Outport  Port=5
  wires:
  Sport/1 -> Data Type Conversion3/1
  Drive/1 -> Data Type Conversion1/1
  Brake/1 -> Data Type Conversion4/1
  Park/1 -> Data Type Conversion5/1
  Reverse/1 -> Data Type Conversion2/1
  Data Type Conversion1/1 -> SwitchDOut/1
  Data Type Conversion2/1 -> SwitchROut/1
  Data Type Conversion3/1 -> SportOut/1
  Data Type Conversion4/1 -> BrakeOut/1
  Data Type Conversion5/1 -> ParkOut/1

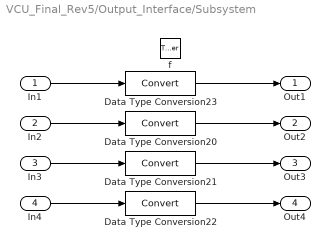
== system VCU_Final_Rev5/Output_Interface/Subsystem ==
  In1 : Inport
  In2 : Inport  Port=2
  In3 : Inport  Port=3
  In4 : Inport  Port=4
  f : TriggerPort  TriggerType=function-call  VariantControl=(inherit)
  Data Type Conversion{20..23} (4 alike) : DataTypeConversion
  Out1 : Outport
  Out2 : Outport  Port=2
  Out3 : Outport  Port=3
  Out4 : Outport  Port=4
  wires:
  Data Type Conversion21/1 -> Out3/1
  Data Type Conversion20/1 -> Out2/1
  In2/1 -> Data Type Conversion20/1
  In1/1 -> Data Type Conversion23/1
  In3/1 -> Data Type Conversion21/1
  In4/1 -> Data Type Conversion22/1
  Data Type Conversion23/1 -> Out1/1
  Data Type Conversion22/1 -> Out4/1

== system VCU_Final_Rev5/PedalInput/Subsystem ==
  ADC2VoltSgl : CoderSF_BSW_Libs/ADC/Read Float ADC Volt  channel=0  voltType=Volt_0_5V  adType=12Bit  ratioV=1  voltRef=5
  Data Type Conversion : DataTypeConversion
  sigInLinkDrvPedacc_volt1 : Outport
  wires:
  Data Type Conversion/1 -> sigInLinkDrvPedacc_volt1/1  "sigInLinkDrvPedacc1_volt"
  ADC2VoltSgl/1 -> Data Type Conversion/1

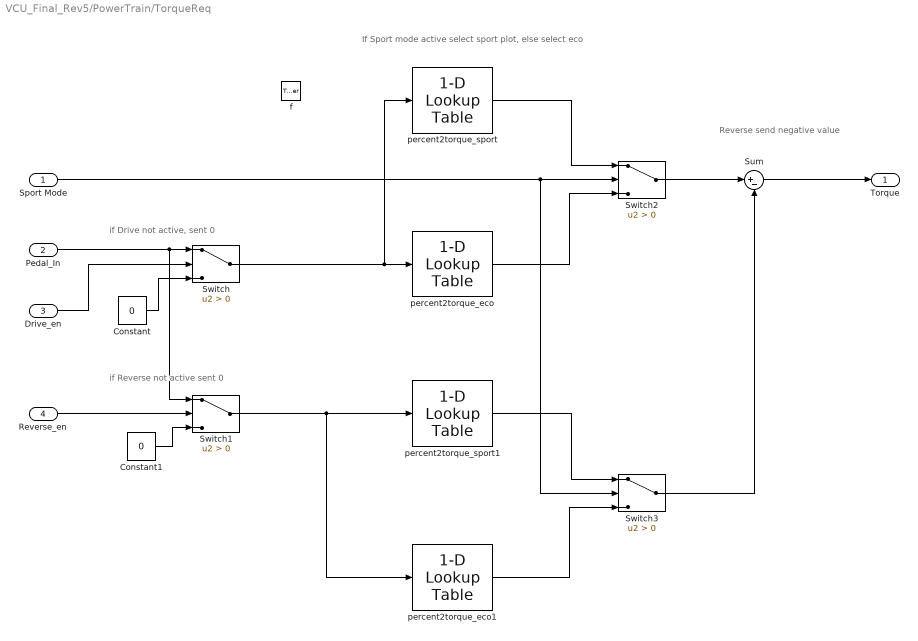
== system VCU_Final_Rev5/PowerTrain/TorqueReq ==
  note: Reverse send
      | negative value
  note: If Sport mode active select sport plot, else select eco
  note: if Reverse not active sent 0
  note: if Drive not active, sent 0
  Sport Mode : Inport
  Pedal_In : Inport  Port=2
  Drive_en : Inport  Port=3
  Reverse_en : Inport  Port=4
  f : TriggerPort  TriggerType=function-call  VariantControl=(inherit)
  Constant : Constant  Value=0
  Constant1 : Constant  Value=0
  Sum : Sum  Inputs=|+-
  Switch{,1..3} (4 alike) : Switch  Criteria=u2 > Threshold
  percent2torque_eco : CoderSF_BSW_Libs/Calibration & Measurement/1-D Lookup Table  nam=percent2torque_eco  breakpoint_type=single  breakpoint_data=[0 100]  table_type=single  table_data=[0 50]
  percent2torque_eco1 : CoderSF_BSW_Libs/Calibration & Measurement/1-D Lookup Table  nam=percent2torque_eco  breakpoint_type=single  breakpoint_data=[0 100]  table_type=single  table_data=[0 50]
  percent2torque_sport : CoderSF_BSW_Libs/Calibration & Measurement/1-D Lookup Table  nam=percent2torque_sport  breakpoint_type=single  breakpoint_data=[0 100]  table_type=single  table_data=[0 200]
  percent2torque_sport1 : CoderSF_BSW_Libs/Calibration & Measurement/1-D Lookup Table  nam=percent2torque_sport  breakpoint_type=single  breakpoint_data=[0 100]  table_type=single  table_data=[0 200]
  Torque : Outport
  wires:
  Sport Mode/1 -> Switch3/2, Switch2/2
  percent2torque_eco/1 -> Switch2/3
  percent2torque_sport/1 -> Switch2/1
  Constant/1 -> Switch/3
  Drive_en/1 -> Switch/2
  Switch/1 -> percent2torque_sport/1, percent2torque_eco/1
  Switch2/1 -> Sum/1
  Constant1/1 -> Switch1/3
  Pedal_In/1 -> Switch1/1, Switch/1
  Switch1/1 -> percent2torque_eco1/1, percent2torque_sport1/1
  Sum/1 -> Torque/1
  percent2torque_eco1/1 -> Switch3/3
  Switch3/1 -> Sum/2
  percent2torque_sport1/1 -> Switch3/1
  Reverse_en/1 -> Switch1/2

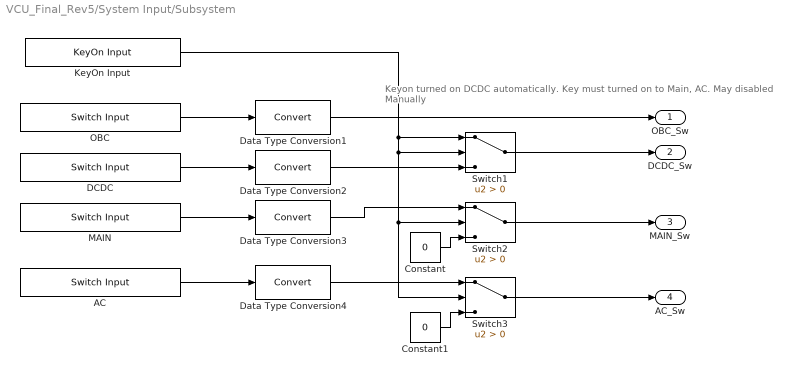
== system VCU_Final_Rev5/System Input/Subsystem ==
  note: Keyon turned on DCDC automatically.
      | Key must turned on to Main,  AC. May disabled Manually
  AC : CoderSF_BSW_Libs/Digital I//O/Switch Input  portNum=DI14
  Constant : Constant  Value=0
  Constant1 : Constant  Value=0
  DCDC : CoderSF_BSW_Libs/Digital I//O/Switch Input  portNum=DI12
  Data Type Conversion{1..4} (4 alike) : DataTypeConversion
  KeyOn Input : CoderSF_BSW_Libs/Digital I//O/KeyOn Input  portNum=DI_KEYON  facAd2Volt=109/27846  uKeyOffThrSet=1  uKeyOnHystSet=1
  MAIN : CoderSF_BSW_Libs/Digital I//O/Switch Input  portNum=DI13
  OBC : CoderSF_BSW_Libs/Digital I//O/Switch Input  portNum=DI10
  Switch1 : Switch  Criteria=u2 > Threshold
  Switch2 : Switch  Criteria=u2 > Threshold
  Switch3 : Switch  Criteria=u2 > Threshold
  OBC_Sw : Outport
  DCDC_Sw : Outport  Port=2
  MAIN_Sw : Outport  Port=3
  AC_Sw : Outport  Port=4
  wires:
  MAIN/1 -> Data Type Conversion3/1
  OBC/1 -> Data Type Conversion1/1
  AC/1 -> Data Type Conversion4/1
  DCDC/1 -> Data Type Conversion2/1
  Data Type Conversion1/1 -> OBC_Sw/1
  Switch1/1 -> DCDC_Sw/1
  Data Type Conversion2/1 -> Switch1/3
  Data Type Conversion4/1 -> Switch3/1
  KeyOn Input/1 -> Switch1/1, Switch3/2, Switch2/2, Switch1/2
  Switch2/1 -> MAIN_Sw/1
  Data Type Conversion3/1 -> Switch2/1
  Constant/1 -> Switch2/3
  Constant1/1 -> Switch3/3
  Switch3/1 -> AC_Sw/1

== system VCU_Final_Rev5/volt2percent/Subsystem ==
  note: Max 100, min 0
  In1 : Inport
  1-D Lookup Table : CoderSF_BSW_Libs/Calibration & Measurement/1-D Lookup Table  nam=throttle_map  breakpoint_type=single  breakpoint_data=[0.3 4.7]  table_type=single  table_data=[0 100]
  Saturation : Saturate  UpperLimit=4.7  LowerLimit=0.3
  Out1 : Outport
  wires:
  In1/1 -> Saturation/1
  1-D Lookup Table/1 -> Out1/1
  Saturation/1 -> 1-D Lookup Table/1
